simulink model "qCAS_v2019b"  (R2019b)
settings: Solver=VariableStepAuto  StartTime=0.0  StopTime=600  RelTol=1e-3
undefined symbols (not defined in the file or in its folder): DiscIntNeverNeededParam, Ts
libraries: simulink x6, rllib x2
settings Model: NumberOfSteps=50  Creator=Daniel A. Udekwe  LastModifiedBy=Daniel A. Udekwe
settings DebuggingCC: SFMachineParentedDataDiag=error

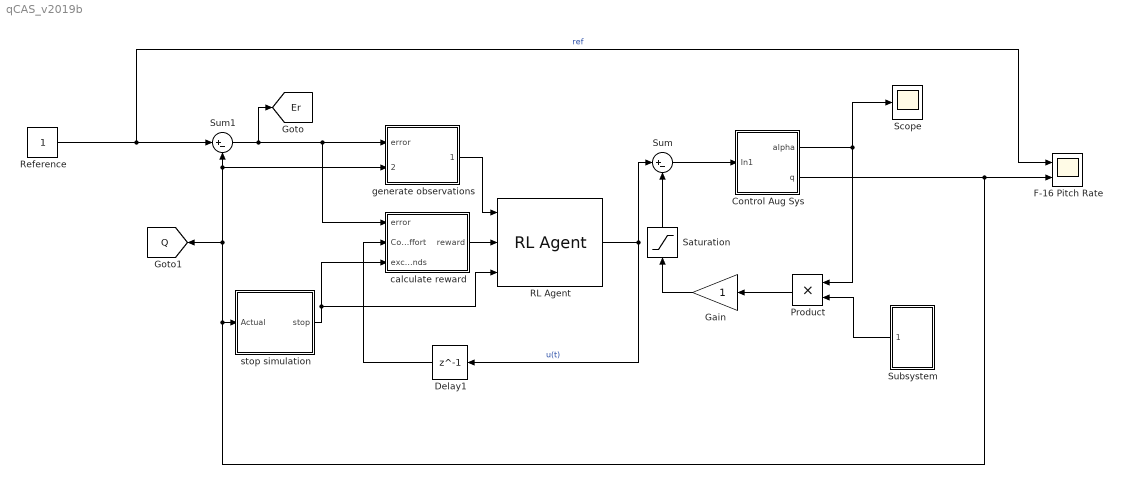
== system qCAS_v2019b ==
  Control Aug Sys : Subsystem
  Delay1 : Delay  DelayLength=1
  F-16 Pitch Rate : Scope  NumInputPorts=2
  Gain : Gain
  Product : Product
  RL Agent : rllib/RL Agent  Agent=agent1  ExternalActionAsInput=off  ProvideCumRwd=off  TreatAsDirectFeedthrough=on
  Reference : Constant
  Saturation : Saturate  UpperLimit=1  LowerLimit=-1
  Scope : Scope
  Subsystem : Subsystem
  Sum : Sum  Inputs=|+-
  Sum1 : Sum  Inputs=|+-  SaturateOnIntegerOverflow=on
  calculate reward : Subsystem
  generate observations : Subsystem
  stop simulation : Subsystem
  tag scope: Er=global, Q=global
  wires:
  RL Agent/1 -> Delay1/1, Sum/1  "u(t)"
  generate observations/1(observations) -> RL Agent/1
  Sum1/1 -> calculate reward/1(error), generate observations/1(error), [Er]
  calculate reward/1(reward) -> RL Agent/2
  Delay1/1 -> calculate reward/2(Control effort)
  stop simulation/1(stop) -> calculate reward/3(exceeds bounds), RL Agent/3
  Control Aug Sys/1(alpha) -> Product/1, Scope/1
  Gain/1 -> Saturation/1
  Control Aug Sys/2(q) -> stop simulation/1(Actual), generate observations/2(pitch rate), Sum1/2, [Q], F-16 Pitch Rate/2
  Product/1 -> Gain/1
  Saturation/1 -> Sum/2
  Reference/1 -> F-16 Pitch Rate/1, Sum1/1  "ref"
  Sum/1 -> Control Aug Sys/1(In1)
  Subsystem/1(action) -> Product/2

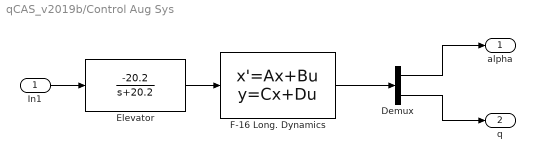
== system qCAS_v2019b/Control Aug Sys ==
  In1 : Inport
  Demux : Demux  Outputs=2
  Elevator : TransferFcn  Numerator=[-20.2]  Denominator=[1 20.2]
  F-16 Long. Dynamics : StateSpace  A=[-0.022 -1.395 -9.828 -0.672; -0.002 -0.582 0 0.908; 0 0 0 1; 3e-7 0.324 0 -0.708]  B=[-1.139; -0.072; 0; -4.301]  C=[0 0 0 1; 0 1 0 0]  D=[0; 0]  InitialCondition=0
  alpha : Outport
  q : Outport  Port=2
  wires:
  F-16 Long. Dynamics/1 -> Demux/1
  Demux/1 -> alpha/1
  Demux/2 -> q/1
  In1/1 -> Elevator/1
  Elevator/1 -> F-16 Long. Dynamics/1

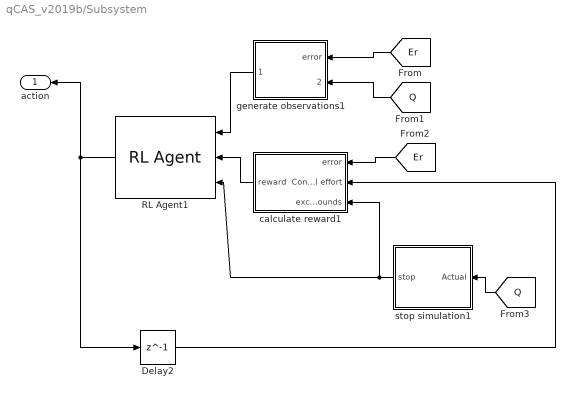
== system qCAS_v2019b/Subsystem ==
  Delay2 : Delay  DelayLength=1
  RL Agent1 : rllib/RL Agent  Agent=agent2  ExternalActionAsInput=off  ProvideCumRwd=off  TreatAsDirectFeedthrough=on
  calculate reward1 : Subsystem
  generate observations1 : Subsystem
  stop simulation1 : Subsystem
  action : Outport
  wires:
  [Er] -> generate observations1/1(error)
  Delay2/1 -> calculate reward1/2(Control effort)
  generate observations1/1(observations) -> RL Agent1/1
  stop simulation1/1(stop) -> calculate reward1/3(exceeds bounds), RL Agent1/3
  calculate reward1/1(reward) -> RL Agent1/2
  RL Agent1/1 -> action/1, Delay2/1
  [Q] -> generate observations1/2(pitch rate)
  [Er] -> calculate reward1/1(error)
  [Q] -> stop simulation1/1(Actual)

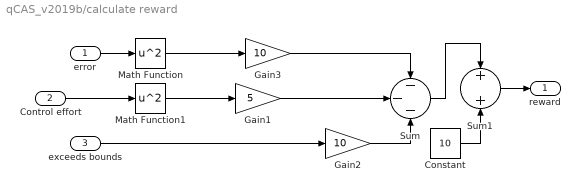
== system qCAS_v2019b/calculate reward ==
  error : Inport
  Control effort : Inport  Port=2
  exceeds bounds : Inport  Port=3
  Constant : Constant  Value=10
  Gain1 : Gain  Gain=5
  Gain2 : Gain  Gain=10
  Gain3 : Gain  Gain=10
  Math Function : Math  Operator=square  SaturateOnIntegerOverflow=on
  Math Function1 : Math  Operator=square  SaturateOnIntegerOverflow=on
  Sum : Sum  Inputs=---  OutDataTypeStr=double
  Sum1 : Sum  OutDataTypeStr=double
  reward : Outport  VectorParamsAs1DForOutWhenUnconnected=off
  wires:
  exceeds bounds/1 -> Gain2/1
  error/1 -> Math Function/1
  Math Function/1 -> Gain3/1
  Gain3/1 -> Sum/1
  Sum/1 -> Sum1/1
  Constant/1 -> Sum1/2
  Sum1/1 -> reward/1
  Math Function1/1 -> Gain1/1
  Gain2/1 -> Sum/3
  Control effort/1 -> Math Function1/1
  Gain1/1 -> Sum/2

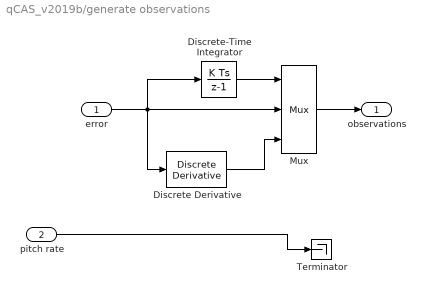
== system qCAS_v2019b/generate observations ==
  error : Inport
  pitch rate : Inport  Port=2
  Discrete Derivative : simulink/Discrete/Discrete Derivative  gainval=1.0  ICPrevScaledInput=0.0  OutMin=[]  OutMax=[]  OutDataType=fixdt(1, 16)  OutScaling=2^-10  DoSatur=off
  Discrete-Time Integrator : DiscreteIntegrator  SampleTime=Ts  ICPrevOutput=DiscIntNeverNeededParam  ICPrevScaledInput=DiscIntNeverNeededParam
  Mux : Mux  Inputs=3
  Terminator : Terminator
  observations : Outport  VectorParamsAs1DForOutWhenUnconnected=off
  wires:
  Discrete-Time Integrator/1 -> Mux/1
  Mux/1 -> observations/1
  pitch rate/1 -> Terminator/1
  error/1 -> Discrete Derivative/1, Mux/2, Discrete-Time Integrator/1
  Discrete Derivative/1 -> Mux/3

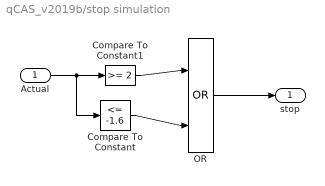
== system qCAS_v2019b/stop simulation ==
  Actual : Inport
  Compare To Constant : simulink/Logic and Bit Operations/Compare To Constant  relop=<=  const=-1.6  OutDataTypeStr=boolean
  Compare To Constant1 : simulink/Logic and Bit Operations/Compare To Constant  relop=>=  const=2  OutDataTypeStr=boolean
  OR : Logic  Operator=OR  IconShape=distinctive  AllPortsSameDT=off  OutDataTypeStr=boolean
  stop : Outport  VectorParamsAs1DForOutWhenUnconnected=off
  wires:
  Compare To Constant1/1 -> OR/1
  Actual/1 -> Compare To Constant/1, Compare To Constant1/1
  Compare To Constant/1 -> OR/2
  OR/1 -> stop/1

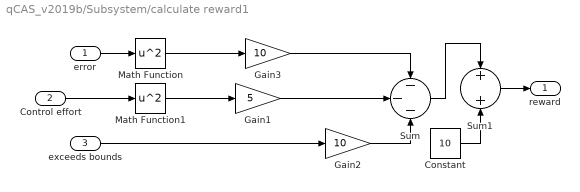
== system qCAS_v2019b/Subsystem/calculate reward1 ==
  error : Inport
  Control effort : Inport  Port=2
  exceeds bounds : Inport  Port=3
  Constant : Constant  Value=10
  Gain1 : Gain  Gain=5
  Gain2 : Gain  Gain=10
  Gain3 : Gain  Gain=10
  Math Function : Math  Operator=square  SaturateOnIntegerOverflow=on
  Math Function1 : Math  Operator=square  SaturateOnIntegerOverflow=on
  Sum : Sum  Inputs=---  OutDataTypeStr=double
  Sum1 : Sum  OutDataTypeStr=double
  reward : Outport  VectorParamsAs1DForOutWhenUnconnected=off
  wires:
  exceeds bounds/1 -> Gain2/1
  error/1 -> Math Function/1
  Math Function/1 -> Gain3/1
  Gain3/1 -> Sum/1
  Sum/1 -> Sum1/1
  Constant/1 -> Sum1/2
  Sum1/1 -> reward/1
  Math Function1/1 -> Gain1/1
  Gain2/1 -> Sum/3
  Control effort/1 -> Math Function1/1
  Gain1/1 -> Sum/2

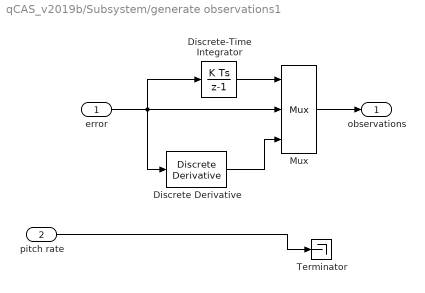
== system qCAS_v2019b/Subsystem/generate observations1 ==
  error : Inport
  pitch rate : Inport  Port=2
  Discrete Derivative : simulink/Discrete/Discrete Derivative  gainval=1.0  ICPrevScaledInput=0.0  OutMin=[]  OutMax=[]  OutDataType=fixdt(1, 16)  OutScaling=2^-10  DoSatur=off
  Discrete-Time Integrator : DiscreteIntegrator  SampleTime=Ts  ICPrevOutput=DiscIntNeverNeededParam  ICPrevScaledInput=DiscIntNeverNeededParam
  Mux : Mux  Inputs=3
  Terminator : Terminator
  observations : Outport  VectorParamsAs1DForOutWhenUnconnected=off
  wires:
  Discrete Derivative/1 -> Mux/3
  error/1 -> Discrete-Time Integrator/1, Mux/2, Discrete Derivative/1
  pitch rate/1 -> Terminator/1
  Mux/1 -> observations/1
  Discrete-Time Integrator/1 -> Mux/1

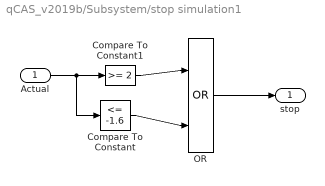
== system qCAS_v2019b/Subsystem/stop simulation1 ==
  Actual : Inport
  Compare To Constant : simulink/Logic and Bit Operations/Compare To Constant  relop=<=  const=-1.6  OutDataTypeStr=boolean
  Compare To Constant1 : simulink/Logic and Bit Operations/Compare To Constant  relop=>=  const=2  OutDataTypeStr=boolean
  OR : Logic  Operator=OR  IconShape=distinctive  AllPortsSameDT=off  OutDataTypeStr=boolean
  stop : Outport  VectorParamsAs1DForOutWhenUnconnected=off
  wires:
  Compare To Constant1/1 -> OR/1
  Actual/1 -> Compare To Constant/1, Compare To Constant1/1
  Compare To Constant/1 -> OR/2
  OR/1 -> stop/1
